simulink model "oving2"  (R2024b)
settings: Solver=ode2  StartTime=0.0  StopTime=100  FixedStep=0.01  RelTol=1e-9  AbsTol=1e-9
undefined symbols (not defined in the file or in its folder): a, b, c, d, f, g, h, i, j, k, l, m, n, o, p
libraries: simulink x17, mylib x1
settings Model: Creator=tormod  LastModifiedBy=jorgen
settings DebuggingCC: UnconnectedInputMsg=warning  UnconnectedOutputMsg=warning  UnconnectedLineMsg=warning
settings ModelReferenceCC: EnableRefExpFcnMdlSchedulingChecks=on
settings RTWCC: GPUComputeCapability=3.5  DLArmComputeVersion=19.05

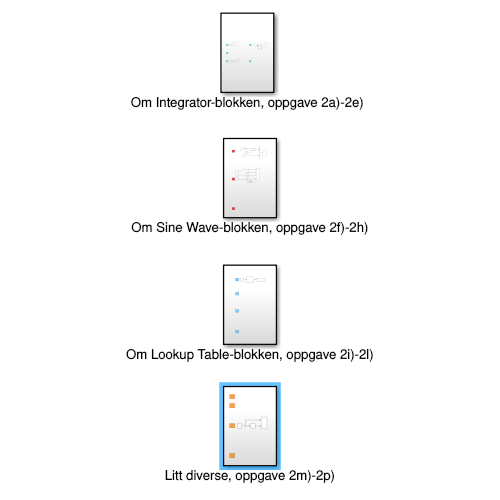
[thumbnail: Simulink's stored preview of the top-level diagram]
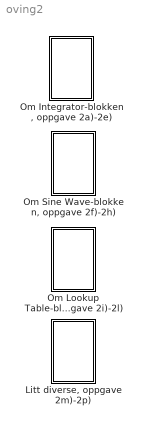
== system oving2 ==
  "Litt diverse, oppgave 2m)-2p)" : Subsystem
  "Om Integrator-blokken, oppgave 2a)-2e)" : Subsystem
  "Om Lookup Table-blokken, oppgave 2i)-2l)" : Subsystem
  "Om Sine Wave-blokken, oppgave 2f)-2h)" : Subsystem

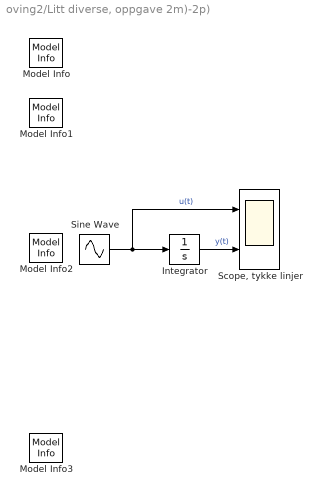
== system oving2/Litt diverse, oppgave 2m)-2p) ==
  Integrator : Integrator  InitialCondition=-0.5/0.3
      settings: AttributesFormatString=IC = %<InitialCondition>
  Model Info : simulink/Model-Wide Utilities/Model Info  Frame=on  DisplayStringWithTags=m)  HorizontalTextAlignment=Center  LeftAlignmentValue=0.5
  Model Info1 : simulink/Model-Wide Utilities/Model Info  Frame=on  DisplayStringWithTags=n)  HorizontalTextAlignment=Center  LeftAlignmentValue=0.5
  Model Info2 : simulink/Model-Wide Utilities/Model Info  Frame=on  DisplayStringWithTags=o)  HorizontalTextAlignment=Center  LeftAlignmentValue=0.5
  Model Info3 : simulink/Model-Wide Utilities/Model Info  Frame=on  DisplayStringWithTags=p)  HorizontalTextAlignment=Center  LeftAlignmentValue=0.5
  "Scope, tykke linjer" : Scope  NumInputPorts=2
  Sine Wave : Sin  Amplitude=0.5  Frequency=0.3  SampleTime=0
      settings: AttributesFormatString=u(t) = %<Amplitude> sin(%<Frequency>t + %<Phase>) + %<Bias>
  wires:
  Sine Wave/1 -> "Scope, tykke linjer"/1, Integrator/1  "u(t)"
  Integrator/1 -> "Scope, tykke linjer"/2  "y(t)"

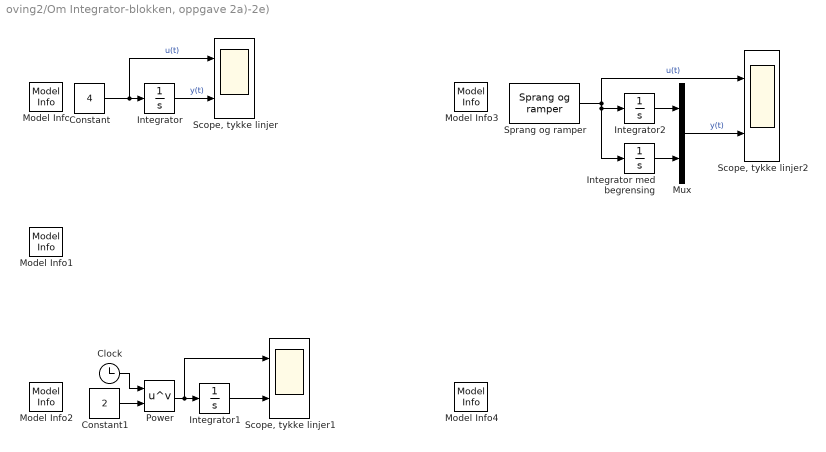
== system oving2/Om Integrator-blokken, oppgave 2a)-2e) ==
  Clock : Clock
  Constant : Constant  Value=4
  Constant1 : Constant  Value=2
  Integrator : Integrator
      settings: AttributesFormatString=IC = %<InitialCondition>
  Integrator med begrensing : Integrator  InitialCondition=40  LimitOutput=on  UpperSaturationLimit=30  LowerSaturationLimit=0
      settings: AttributesFormatString=|
      | IC = %<InitialCondition>
      | Max = %<UpperSaturationLimit>
      | Min = %<LowerSaturationLimit>
  Integrator1 : Integrator
      settings: AttributesFormatString=IC = %<InitialCondition>
  Integrator2 : Integrator  InitialCondition=10
      settings: AttributesFormatString=IC = %<InitialCondition>
  Model Info : simulink/Model-Wide Utilities/Model Info  Frame=on  DisplayStringWithTags=a)  HorizontalTextAlignment=Center  LeftAlignmentValue=0.5
  Model Info1 : simulink/Model-Wide Utilities/Model Info  Frame=on  DisplayStringWithTags=b)  HorizontalTextAlignment=Center  LeftAlignmentValue=0.5
  Model Info2 : simulink/Model-Wide Utilities/Model Info  Frame=on  DisplayStringWithTags=c)  HorizontalTextAlignment=Center  LeftAlignmentValue=0.5
  Model Info3 : simulink/Model-Wide Utilities/Model Info  Frame=on  DisplayStringWithTags=d)  HorizontalTextAlignment=Center  LeftAlignmentValue=0.5
  Model Info4 : simulink/Model-Wide Utilities/Model Info  Frame=on  DisplayStringWithTags=e)  HorizontalTextAlignment=Center  LeftAlignmentValue=0.5
  Mux : Mux  Inputs=2
  Power : Math  Operator=pow
  "Scope, tykke linjer" : Scope  NumInputPorts=2
  "Scope, tykke linjer1" : Scope  NumInputPorts=2
  "Scope, tykke linjer2" : Scope  NumInputPorts=2
  Sprang og ramper : mylib/ELE130/Sprang og ramper  tidspunkt=[0 3 9 17 20]  utgangsverdi=[0 6 -8 4 0]  valg=Trappetrinn
      settings: SourceProductName=Eget bibliotek
      settings: AttributesFormatString=|
      | t = %<tidspunkt>
      | u = %<utgangsverdi>
  wires:
  Constant/1 -> "Scope, tykke linjer"/1, Integrator/1  "u(t)"
  Integrator/1 -> "Scope, tykke linjer"/2  "y(t)"
  Clock/1 -> Power/1
  Constant1/1 -> Power/2
  Power/1 -> "Scope, tykke linjer1"/1, Integrator1/1
  Integrator1/1 -> "Scope, tykke linjer1"/2
  Integrator2/1 -> Mux/1
  Integrator med begrensing/1 -> Mux/2
  Sprang og ramper/1 -> Integrator med begrensing/1, Integrator2/1, "Scope, tykke linjer2"/1  "u(t)"
  Mux/1 -> "Scope, tykke linjer2"/2  "y(t)"

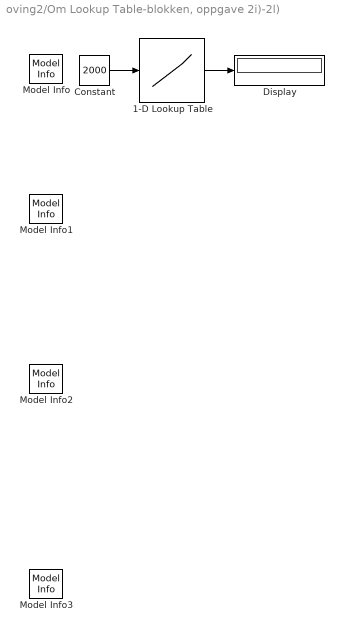
== system oving2/Om Lookup Table-blokken, oppgave 2i)-2l) ==
  1-D Lookup Table : Lookup_n-D  NumberOfTableDimensions=1  LookupTableObject=T  BreakpointsForDimension1=[-150, -100, -50, -0.001, 0, 2, 4, 6, 8, 10, 30, 50, 70, 100]  Table=[932.5, 930, 923.75, 915, 1000, 999.9, 999.8, 999.6, 999.4, 999, 995, 987.5, 977.5, 958 ]  InternalRulePriority=Speed  RndMeth=Simplest
      settings: AttributesFormatString=|
      | INN = %<BreakpointsForDimension1>
      | UT = %<Table>
  Constant : Constant  Value=2000
  Display : Display
      settings: Decimation=3
  Model Info : simulink/Model-Wide Utilities/Model Info  Frame=on  DisplayStringWithTags=i)  HorizontalTextAlignment=Center  LeftAlignmentValue=0.5
  Model Info1 : simulink/Model-Wide Utilities/Model Info  Frame=on  DisplayStringWithTags=j)  HorizontalTextAlignment=Center  LeftAlignmentValue=0.5
  Model Info2 : simulink/Model-Wide Utilities/Model Info  Frame=on  DisplayStringWithTags=k)  HorizontalTextAlignment=Center  LeftAlignmentValue=0.5
  Model Info3 : simulink/Model-Wide Utilities/Model Info  Frame=on  DisplayStringWithTags=l)  HorizontalTextAlignment=Center  LeftAlignmentValue=0.5
  wires:
  Constant/1 -> 1-D Lookup Table/1
  1-D Lookup Table/1 -> Display/1

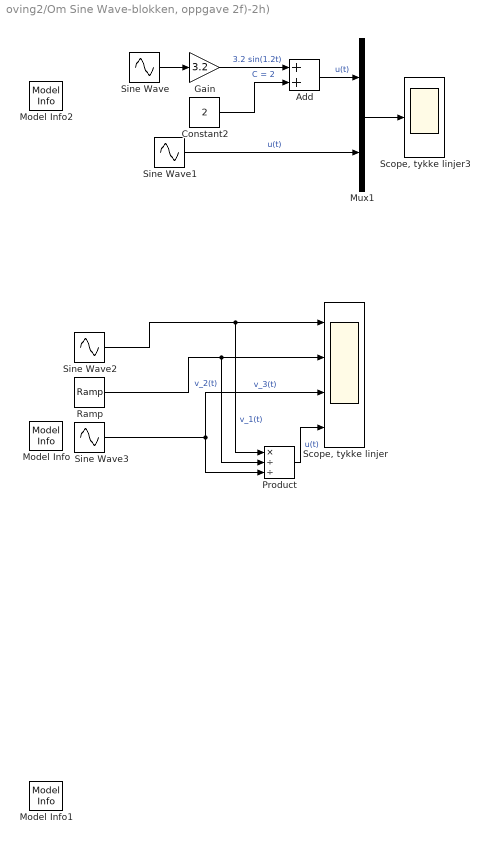
== system oving2/Om Sine Wave-blokken, oppgave 2f)-2h) ==
  Add : Sum
  Constant2 : Constant  Value=2
  Gain : Gain  Gain=3.2
  Model Info : simulink/Model-Wide Utilities/Model Info  Frame=on  DisplayStringWithTags=g)  HorizontalTextAlignment=Center  LeftAlignmentValue=0.5
  Model Info1 : simulink/Model-Wide Utilities/Model Info  Frame=on  DisplayStringWithTags=h)  HorizontalTextAlignment=Center  LeftAlignmentValue=0.5
  Model Info2 : simulink/Model-Wide Utilities/Model Info  Frame=on  DisplayStringWithTags=f)  HorizontalTextAlignment=Center  LeftAlignmentValue=0.5
  Mux1 : Mux  Inputs=2
  Product : Product  Inputs=*//
  Ramp : simulink/Sources/Ramp  slope=0.3  start=15  InitialOutput=1
      settings: AttributesFormatString="u(t) = %<InitialOutput>  + %<slope> (t - %<start>)"
  "Scope, tykke linjer" : Scope  NumInputPorts=4
  "Scope, tykke linjer3" : Scope
  Sine Wave : Sin  Frequency=1.2  SampleTime=0
      settings: AttributesFormatString=u(t) = %<Amplitude> sin(%<Frequency>t + %<Phase>) + %<Bias>
  Sine Wave1 : Sin  Amplitude=3.2  Bias=2  Frequency=1.2  SampleTime=0
      settings: AttributesFormatString=u(t) = %<Amplitude> sin(%<Frequency>t + %<Phase>) + %<Bias>
  Sine Wave2 : Sin  Amplitude=3.2  Bias=2  Frequency=1.2  SampleTime=0
      settings: AttributesFormatString=u(t) = %<Amplitude> sin(%<Frequency>t + %<Phase>) + %<Bias>
  Sine Wave3 : Sin  Amplitude=1.7  Bias=3  Frequency=0.7  Phase=pi/2  SampleTime=0
      settings: AttributesFormatString=u(t) = %<Amplitude> sin(%<Frequency>t + %<Phase>) + %<Bias>
  wires:
  Gain/1 -> Add/1  "3.2 sin(1.2t)"
  Sine Wave/1 -> Gain/1
  Sine Wave1/1 -> Mux1/2  "u(t)"
  Mux1/1 -> "Scope, tykke linjer3"/1
  Add/1 -> Mux1/1  "u(t)"
  Constant2/1 -> Add/2  "C = 2"
  Ramp/1 -> Product/2, "Scope, tykke linjer"/2  "v_2(t)"
  Sine Wave2/1 -> Product/1, "Scope, tykke linjer"/1  "v_1(t)"
  Sine Wave3/1 -> "Scope, tykke linjer"/3, Product/3  "v_3(t)"
  Product/1 -> "Scope, tykke linjer"/4  "u(t)"
